simulink subsystem "ServoMotor"  (R2024b)
settings: Solver=VariableStepAuto  StartTime=0.0  StopTime=10.0  RelTol=1e-3
values from neighbouring files (symbols this model uses):
  a = 0.1    [matlab.mat]    (also in params.mat)
  J = 1    [matlab.mat]    (also in params.mat)
  K = 0.1    [matlab.mat]    (also in params.mat)
  Kf = 0.1    [matlab.mat]    (also in params.mat)
settings Model: Creator=mohammedazab  LastModifiedBy=mohammedazab

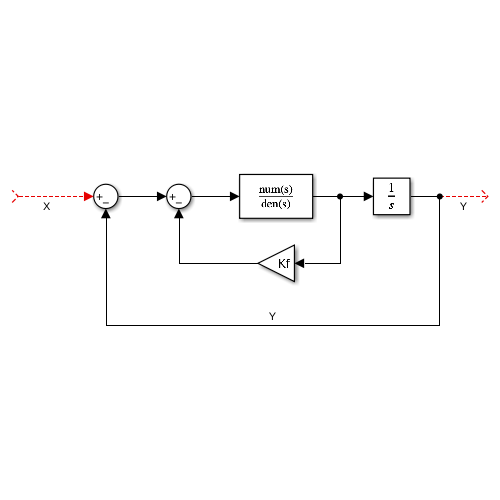
[thumbnail: Simulink's stored preview of the top-level diagram]
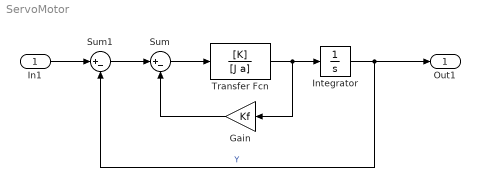
== system ServoMotor ==
  In1 : Inport
  Gain : Gain  Gain=Kf
  Integrator : Integrator
  Sum : Sum  Inputs=|+-
  Sum1 : Sum  Inputs=|+-
  Transfer Fcn : TransferFcn  Numerator=[K]  Denominator=[J a]
  Out1 : Outport
  wires:
  Transfer Fcn/1 -> Gain/1, Integrator/1
  Sum/1 -> Transfer Fcn/1
  Integrator/1 -> Sum1/2, Out1/1  "Y"
  Gain/1 -> Sum/2
  Sum1/1 -> Sum/1
  In1/1 -> Sum1/1
